simulink model "Test_Comm_and_Motion"  (R2018a)
settings: Solver=FixedStepAuto  StartTime=0.0  StopTime=inf  FixedStep=0.00001  RelTol=1e-3
settings Model: Creator=张紫薇  LastModifiedBy=lenovo

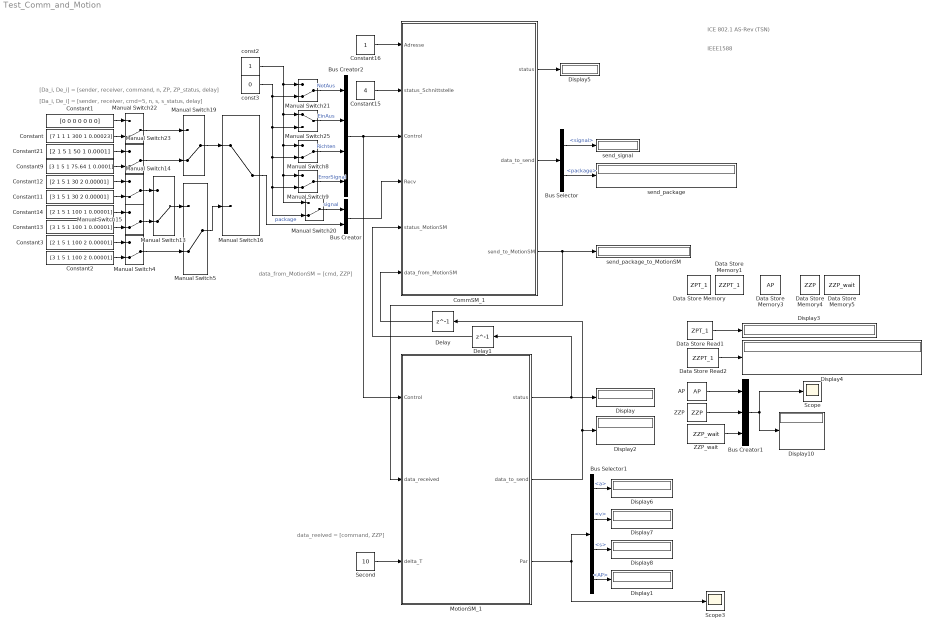
== system Test_Comm_and_Motion ==
  note: IEEE1588
  note: ICE 802.1 AS-Rev (TSN)
  note: data_from_MotionSM = [cmd, ZZP]
  note: [Da_i, De_i] = [sender, receiver, command, n, ZP, ZP_status, delay]
  note: data_reeived = [command, ZZP]
  note: [Da_i, De_i] = [sender, receiver, cmd=5, n, s, s_status, delay]
  AP : DataStoreRead  DataStoreName=AP
  Bus Creator1 : BusCreator  Inputs=3
  Bus Creator : BusCreator  Inputs=2
  Bus Creator2 : BusCreator  Inputs=4
  Bus Selector : BusSelector  OutputSignals=signal,package
  Bus Selector1 : BusSelector  OutputSignals=a,v,s,AP
  CommSM_1 : Subsystem
  Constant : Constant  Value=[7 1 1 1 300 1 0.00023]  OutDataTypeStr=double
  Constant1 : Constant  Value=[0 0 0 0 0 0 0]  OutDataTypeStr=double
  Constant11 : Constant  Value=[3 1 5 1 30 2 0.00001]  OutDataTypeStr=double
  Constant12 : Constant  Value=[2 1 5 1 30 2 0.00001]  OutDataTypeStr=double
  Constant13 : Constant  Value=[3 1 5 1 100 1 0.00001]  OutDataTypeStr=double
  Constant14 : Constant  Value=[2 1 5 1 100 1 0.00001]  OutDataTypeStr=double
  Constant15 : Constant  Value=4  OutDataTypeStr=double
  Constant16 : Constant
  Constant2 : Constant  Value=[3 1 5 1 100 2 0.00001]  OutDataTypeStr=double
  Constant21 : Constant  Value=[2 1 5 1 50 1 0.0001]  OutDataTypeStr=double
  Constant3 : Constant  Value=[2 1 5 1 100 2 0.00001]  OutDataTypeStr=double
  Constant9 : Constant  Value=[3 1 5 1 75.64 1 0.0001]  OutDataTypeStr=double
  Data Store Memory : DataStoreMemory  DataStoreName=ZPT_1  ReadBeforeWriteMsg=warning  WriteAfterWriteMsg=warning  WriteAfterReadMsg=warning  InitialValue=zeros(1,3)  ShowAdditionalParam=off  OutDataTypeStr=double  Dimensions=[1,3]
  Data Store Memory1 : DataStoreMemory  DataStoreName=ZZPT_1  ReadBeforeWriteMsg=warning  WriteAfterWriteMsg=warning  WriteAfterReadMsg=warning  InitialValue=zeros(3,4)  ShowAdditionalParam=off  OutDataTypeStr=double  Dimensions=[3,4]
  Data Store Memory3 : DataStoreMemory  DataStoreName=AP  ReadBeforeWriteMsg=warning  WriteAfterWriteMsg=warning  WriteAfterReadMsg=warning  ShowAdditionalParam=off  OutMin=[0]  OutMax=[100]  OutDataTypeStr=double  Dimensions=1
  Data Store Memory4 : DataStoreMemory  DataStoreName=ZZP  ReadBeforeWriteMsg=warning  WriteAfterWriteMsg=warning  WriteAfterReadMsg=warning  ShowAdditionalParam=off  OutDataTypeStr=double  Dimensions=1
  Data Store Memory5 : DataStoreMemory  DataStoreName=ZZP_wait  ReadBeforeWriteMsg=warning  WriteAfterWriteMsg=warning  WriteAfterReadMsg=warning  ShowAdditionalParam=off  OutDataTypeStr=double  Dimensions=1
  Data Store Read1 : DataStoreRead  DataStoreName=ZPT_1
  Data Store Read2 : DataStoreRead  DataStoreName=ZZPT_1
  Delay : Delay  DelayLength=1
  Delay1 : Delay  DelayLength=1
  Display{,1..8,10} (10 alike) : Display
      Display1 settings: Format=decimal (Stored Integer)
      Display10 settings: Format=decimal (Stored Integer)
      Display8 settings: Format=decimal (Stored Integer)
  Manual Switch{4..5,8..9,13..15,19..23} (12 alike) : ManualSwitch  CurrentSetting=0
  Manual Switch16 : ManualSwitch
  Manual Switch25 : ManualSwitch
  MotionSM_1 : Subsystem
  Scope : Scope
  Scope3 : Scope
  Second : Constant  Value=10
  ZZP : DataStoreRead  DataStoreName=ZZP
  ZZP_wait : DataStoreRead  DataStoreName=ZZP_wait
  const2 : Constant  OutDataTypeStr=boolean
  const3 : Constant  Value=0  OutDataTypeStr=boolean
  send_package : Display
  send_package_to_MotionSM : Display
  send_signal : Display
  wires:
  Manual Switch5/1 -> Manual Switch16/2
  Data Store Read2/1 -> Display4/1
  Manual Switch13/1 -> Manual Switch5/1
  Manual Switch19/1 -> Manual Switch16/1
  Constant3/1 -> Manual Switch4/1
  Delay1/1 -> CommSM_1/5(status_MotionSM)
  Delay/1 -> CommSM_1/6(data_from_MotionSM)
  Constant11/1 -> Manual Switch14/2
  Constant2/1 -> Manual Switch4/2
  const3/1 -> Manual Switch20/2, Manual Switch9/2, Manual Switch8/2, Manual Switch25/2, Manual Switch21/2
  MotionSM_1/1(status) -> Delay1/1, Display/1
  Constant/1 -> Manual Switch22/2
  Data Store Read1/1 -> Display3/1
  Constant1/1 -> Manual Switch22/1
  Bus Selector/1 -> send_signal/1  "<signal>"
  Second/1 -> MotionSM_1/3(delta_T)
  Manual Switch15/1 -> Manual Switch13/2
  Bus Selector/2 -> send_package/1  "<package>"
  Manual Switch4/1 -> Manual Switch5/2
  Constant21/1 -> Manual Switch23/1
  CommSM_1/3(send_to_MotionSM) -> send_package_to_MotionSM/1, MotionSM_1/2(data_received)
  Manual Switch22/1 -> Manual Switch19/1
  Manual Switch14/1 -> Manual Switch13/1
  Bus Selector1/2 -> Display7/1  "<v>"
  Constant14/1 -> Manual Switch15/1
  Constant15/1 -> CommSM_1/2(status_Schnittstelle)
  Bus Selector1/1 -> Display6/1  "<a>"
  Constant12/1 -> Manual Switch14/1
  Constant13/1 -> Manual Switch15/2
  const2/1 -> Manual Switch20/1, Manual Switch9/1, Manual Switch8/1, Manual Switch25/1, Manual Switch21/1
  Constant9/1 -> Manual Switch23/2
  CommSM_1/1(status) -> Display5/1
  MotionSM_1/2(data_to_send) -> Delay/1, Display2/1
  Manual Switch23/1 -> Manual Switch19/2
  Constant16/1 -> CommSM_1/1(Adresse)
  Bus Selector1/3 -> Display8/1  "<s>"
  CommSM_1/2(data_to_send) -> Bus Selector/1
  Manual Switch20/1 -> Bus Creator/1  "signal"
  Manual Switch16/1 -> Bus Creator/2  "package"
  Bus Creator/1 -> CommSM_1/4(Recv)
  MotionSM_1/3(Par) -> Bus Selector1/1, Scope3/1
  ZZP_wait/1 -> Bus Creator1/3
  ZZP/1 -> Bus Creator1/2
  AP/1 -> Bus Creator1/1
  Bus Creator1/1 -> Display10/1, Scope/1
  Bus Selector1/4 -> Display1/1  "<AP>"
  Manual Switch21/1 -> Bus Creator2/1  "NotAus"
  Manual Switch25/1 -> Bus Creator2/2  "EinAus"
  Manual Switch8/1 -> Bus Creator2/3  "Richten"
  Manual Switch9/1 -> Bus Creator2/4  "ErrorSignal"
  Bus Creator2/1 -> MotionSM_1/1(Control), CommSM_1/3(Control)

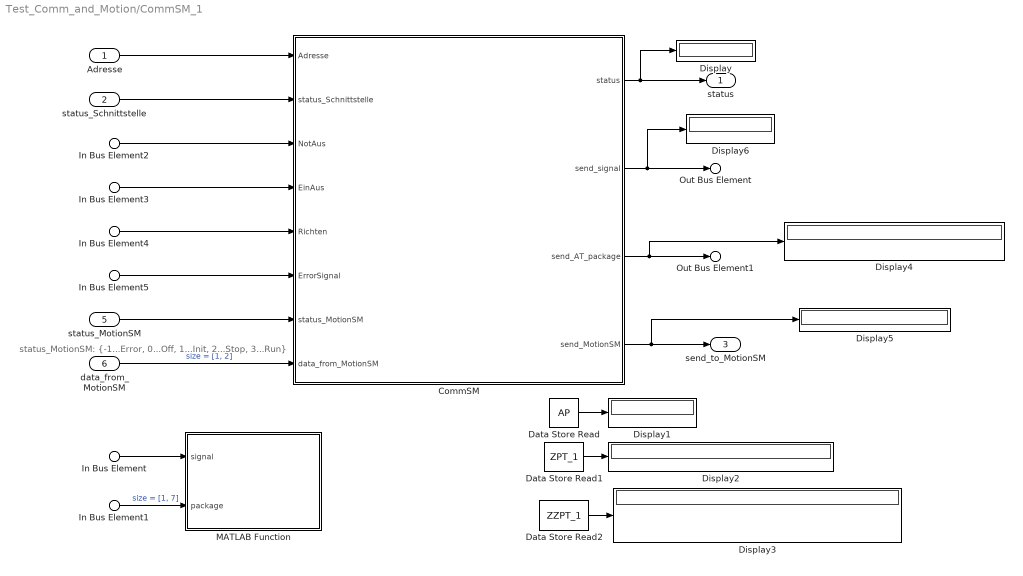
== system Test_Comm_and_Motion/CommSM_1 ==
  note: status_MotionSM: {-1...Error, 0...Off, 1...Init, 2...Stop, 3...Run}
  Adresse : Inport  OutDataTypeStr=double  PortDimensions=1
  status_Schnittstelle : Inport  Port=2  OutDataTypeStr=double  PortDimensions=1
  In Bus Element2 : Inport  Port=3  PortName=Control  Element=NotAus
  In Bus Element3 : Inport  Port=3  PortName=Control  Element=EinAus
  In Bus Element4 : Inport  Port=3  PortName=Control  Element=Richten
  In Bus Element5 : Inport  Port=3  PortName=Control  Element=ErrorSignal
  In Bus Element : Inport  Port=4  PortName=Recv  Element=signal
  In Bus Element1 : Inport  Port=4  PortName=Recv  Element=package
  status_MotionSM : Inport  Port=5  OutDataTypeStr=double  PortDimensions=1
  data_from_MotionSM : Inport  Port=6  OutDataTypeStr=double  PortDimensions=2
  CommSM : Stateflow chart  TreatAsAtomicUnit=on
  Data Store Read : DataStoreRead  DataStoreName=AP
  Data Store Read1 : DataStoreRead  DataStoreName=ZPT_1
  Data Store Read2 : DataStoreRead  DataStoreName=ZZPT_1
  Display{,1..6} (7 alike) : Display
  MATLAB Function : MATLAB Function  TreatAsAtomicUnit=on
  status : Outport  OutDataTypeStr=double  PortDimensions=1
  Out Bus Element : Outport  Port=2  PortName=data_to_send  Element=signal
  Out Bus Element1 : Outport  Port=2  PortName=data_to_send  Element=package
  send_to_MotionSM : Outport  Port=3
  wires:
  In Bus Element2/1 -> CommSM/3(NotAus)
  In Bus Element3/1 -> CommSM/4(EinAus)
  In Bus Element4/1 -> CommSM/5(Richten)
  In Bus Element5/1 -> CommSM/6(ErrorSignal)
  status_Schnittstelle/1 -> CommSM/2(status_Schnittstelle)
  In Bus Element/1 -> MATLAB Function/1(signal)
  In Bus Element1/1 -> MATLAB Function/2(package)  "size = [1, 7]"
  data_from_MotionSM/1 -> CommSM/8(data_from_MotionSM)  "size = [1, 2]"
  status_MotionSM/1 -> CommSM/7(status_MotionSM)
  Adresse/1 -> CommSM/1(Adresse)
  CommSM/1(status) -> Display/1, status/1
  CommSM/3(send_AT_package) -> Out Bus Element1/1, Display4/1
  CommSM/4(send_MotionSM) -> Display5/1, send_to_MotionSM/1
  CommSM/2(send_signal) -> Out Bus Element/1, Display6/1
  Data Store Read/1 -> Display1/1
  Data Store Read1/1 -> Display2/1
  Data Store Read2/1 -> Display3/1

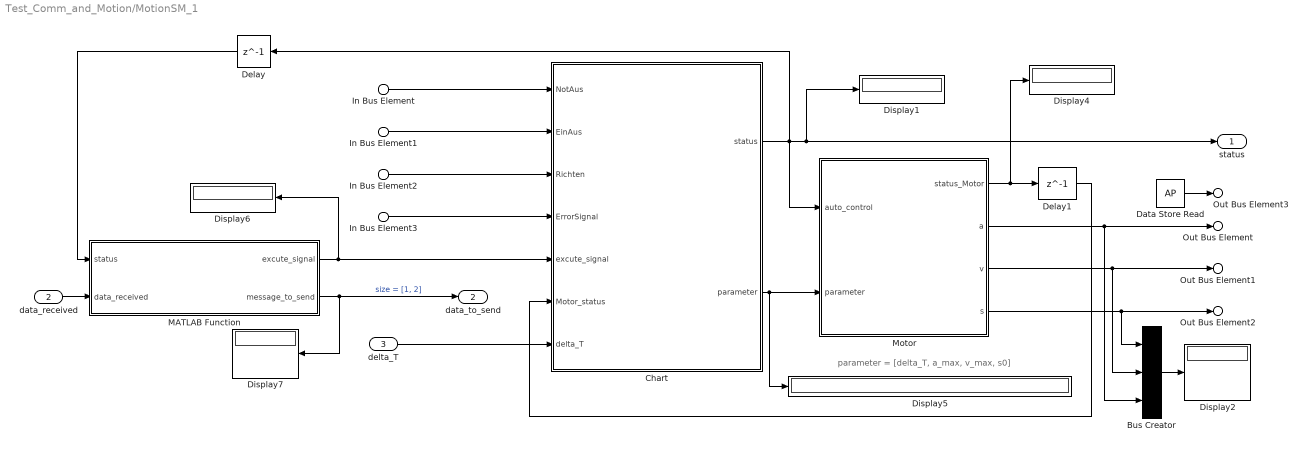
== system Test_Comm_and_Motion/MotionSM_1 ==
  note: parameter = [delta_T, a_max, v_max, s0]
  In Bus Element : Inport  PortName=Control  Element=NotAus
  In Bus Element1 : Inport  PortName=Control  Element=EinAus
  In Bus Element2 : Inport  PortName=Control  Element=Richten
  In Bus Element3 : Inport  PortName=Control  Element=ErrorSignal
  data_received : Inport  Port=2  OutDataTypeStr=double  PortDimensions=2
  delta_T : Inport  Port=3
  Bus Creator : BusCreator  Inputs=3
  Chart : Stateflow chart  TreatAsAtomicUnit=on
  Data Store Read : DataStoreRead  DataStoreName=AP
  Delay : Delay  DelayLength=1
  Delay1 : Delay  DelayLength=1
  Display{1..2,4..7} (6 alike) : Display
  MATLAB Function : MATLAB Function  TreatAsAtomicUnit=on
  Motor : Subsystem
  status : Outport
  data_to_send : Outport  Port=2  OutDataTypeStr=double  PortDimensions=2
  Out Bus Element : Outport  Port=3  PortName=Par  Element=a
  Out Bus Element1 : Outport  Port=3  PortName=Par  Element=v
  Out Bus Element2 : Outport  Port=3  PortName=Par  Element=s
  Out Bus Element3 : Outport  Port=3  PortName=Par  Element=AP
  wires:
  Chart/1(status) -> Motor/1(auto_control), Delay/1, Display1/1, status/1
  In Bus Element1/1 -> Chart/2(EinAus)
  In Bus Element/1 -> Chart/1(NotAus)
  In Bus Element2/1 -> Chart/3(Richten)
  In Bus Element3/1 -> Chart/4(ErrorSignal)
  Motor/1(status_Motor) -> Display4/1, Delay1/1
  data_received/1 -> MATLAB Function/2(data_received)
  Delay1/1 -> Chart/6(Motor_status)
  MATLAB Function/1(excute_signal) -> Chart/5(excute_signal), Display6/1
  MATLAB Function/2(message_to_send) -> Display7/1, data_to_send/1  "size = [1, 2]"
  delta_T/1 -> Chart/7(delta_T)
  Motor/2(a) -> Bus Creator/3, Out Bus Element/1
  Motor/3(v) -> Bus Creator/2, Out Bus Element1/1
  Motor/4(s) -> Bus Creator/1, Out Bus Element2/1
  Chart/2(parameter) -> Motor/2(parameter), Display5/1
  Delay/1 -> MATLAB Function/1(status)
  Data Store Read/1 -> Out Bus Element3/1
  Bus Creator/1 -> Display2/1

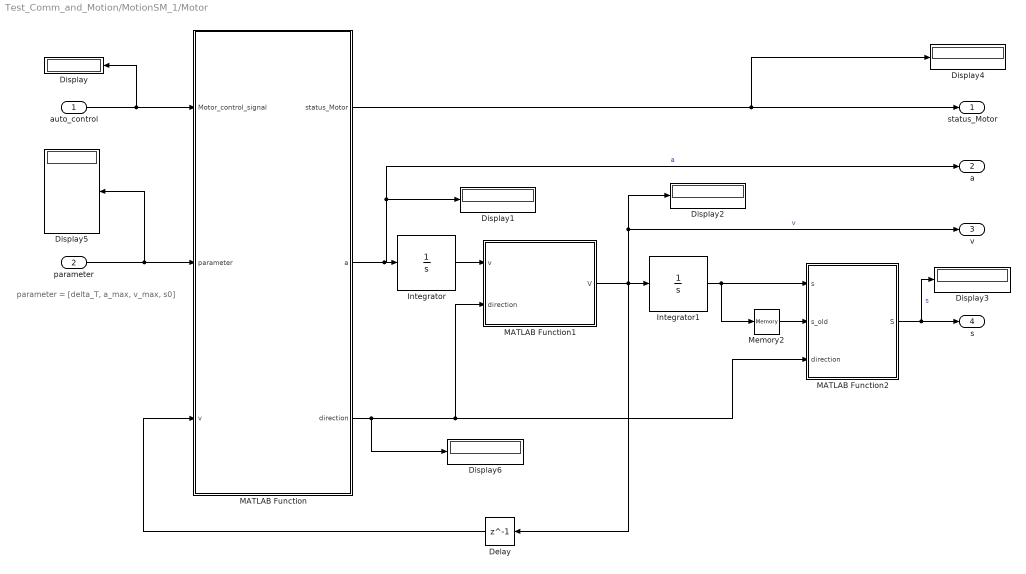
== system Test_Comm_and_Motion/MotionSM_1/Motor ==
  note: parameter = [delta_T, a_max, v_max, s0]
  auto_control : Inport
  parameter : Inport  Port=2
  Delay : Delay  DelayLength=1
  Display{,1..6} (7 alike) : Display
  Integrator : Integrator
  Integrator1 : Integrator
  MATLAB Function : MATLAB Function  TreatAsAtomicUnit=on
  MATLAB Function1 : MATLAB Function  TreatAsAtomicUnit=on
  MATLAB Function2 : MATLAB Function  TreatAsAtomicUnit=on
  Memory2 : Memory
  status_Motor : Outport
  a : Outport  Port=2
  v : Outport  Port=3
  s : Outport  Port=4
  wires:
  Integrator/1 -> MATLAB Function1/1(v)
  Integrator1/1 -> MATLAB Function2/1(s), Memory2/1
  auto_control/1 -> Display/1, MATLAB Function/1(Motor_control_signal)
  MATLAB Function/1(status_Motor) -> Display4/1, status_Motor/1
  parameter/1 -> Display5/1, MATLAB Function/2(parameter)
  MATLAB Function/2(a) -> a/1, Display1/1, Integrator/1  "a"
  MATLAB Function1/1(V) -> Display2/1, v/1, Delay/1, Integrator1/1  "v"
  MATLAB Function/3(direction) -> MATLAB Function1/2(direction), MATLAB Function2/3(direction), Display6/1
  MATLAB Function2/1(S) -> Display3/1, s/1  "s"
  Memory2/1 -> MATLAB Function2/2(s_old)
  Delay/1 -> MATLAB Function/3(v)

== matlab function Test_Comm_and_Motion/MotionSM_1/MATLAB Function ==
  data: status input double size=1; excute_signal output boolean size=1; message_to_send output double size=2; data_received input double size=2; ZZP_wait data_store_memory size=1; AP data_store_memory; ZZP data_store_memory
%data_received / message_to_send = [cmd, ZZP]
%cmd:  1...setP, 2...getP, 3...excP

function [excute_signal, message_to_send] = message_analysis(status, data_received)

global ZZP_wait
global AP
global ZZP

excute_signal = false;

cmd = data_received(1);
message_to_send = [0, 0]';

switch cmd
    case 1      %setP
        excute_signal = false;
        if ((status >= 1) && (status <= 3))
            ZZP_wait = data_received(2);
            message_to_send = [2, ZZP_wait]';
        end
        
    case 3      %excP
        excute_signal = true;
        if ((ZZP == AP) && (status == 2) && (ZZP~=ZZP_wait))
            ZZP = ZZP_wait;
        end
end
end

== matlab function Test_Comm_and_Motion/MotionSM_1/Motor/MATLAB Function ==
  settings: updateMethod=DISCRETE
  data: status_Motor output boolean size=1; Motor_control_signal input double size=1; parameter input double size=4; v input double size=1; a output double size=1; direction output double size=1; AP data_store_memory; ZZP data_store_memory
function [status_Motor, a, direction]= Motor(Motor_control_signal, parameter, v)

%delta_T = parameter(1);
a_max = abs(parameter(2));
v_max = abs(parameter(3));
s0 = parameter(4);
direction = 0;
a = 0;

s_a = 0.5 * v_max * v_max / a_max;
a_bremsen = 100000;     % 100 m/s^2

global AP
global ZZP

switch Motor_control_signal
    case {-1, 0}            %Error & Off
        if v > 0
            a = -a_bremsen;
            direction = 1;
        elseif v < 0
            a = a_bremsen;
            direction = -1;
        else
            a = 0;
            direction = 0;
        end
             
    case 1                  %Init
        if (AP > 0)
            direction = s0;
            if ((ZZP - AP) < (-s_a)) && (v > (-v_max))
                a = -a_max;
            elseif ((ZZP - AP) >= (-s_a)) && (ZZP < AP) && (v < 0)
                a = a_max;
            else
                a = 0;
            end
        else
            a = 0;
            AP = 0;
        end
        
    case 2                  %Stop
        if (v > 0)
            a = -a_max;
            direction = 1;
        elseif (v < 0)
            a = a_max;
            direction = -1;
        else
            a = 0;
            direction = 0;
        end
        
    case 3                  %run
        direction = s0;
        if (s0 > 0)   %forward
            %v_control(2) = s0;
            if ((ZZP - AP) > s_a) && (v < v_max)
                a = a_max;
            elseif ((ZZP - AP) <= s_a) && (ZZP > AP) && (v > 0)
                a = -a_max;
            else
                a = 0;
            end
        end
        if (s0 < 0)    %backward
            if ((ZZP - AP) < (-s_a)) && (v > (-v_max))
                a = -a_max;
            elseif ((ZZP - AP) >= (-s_a)) && (ZZP < AP) && (v < 0)
                a = a_max;
            else
                a = 0;
            end
        end
end
        
%status_Motor: false...Stopped, true...Running
if (a == 0) && (v == 0)
    status_Motor = false;
else
    status_Motor = true;
end

end

== stateflow chart Test_Comm_and_Motion/MotionSM_1/Chart ==
  state Off
    entry: status=0;
  state Init
    entry: status=1; parameter=Par_1(delta_T);
  state On
    state Stop
      entry: status=2;
    state Run
      entry: status=3;
    (default) -> Stop
    Stop -> Run : [excute_signal==1 && ZZP~=AP && Motor_status == 0]
        | {parameter=Par(delta_T)}
    Run -> Stop : [ZZP==AP && ~Motor_status]
  state Error
    entry: status=-1;
  (default) -> Off
  Init -> Off [order 1] : [~EinAus]
  Off -> Init [order 2] : [EinAus && ~ NotAus]{parameter=[delta_T,0,0,0]'}
  Init -> Error [order 2] : [Motor_status==-1 || NotAus || ErrorSignal]
  Off -> Error [order 1] : [EinAus && (ErrorSignal || NotAus)]
  Error -> Off [order 1] : [~EinAus]
  On -> Off [order 1] : [~EinAus]
  Error -> Init [order 2] : [Richten]{parameter=[delta_T,0,0,0]'}
  Init -> On [order 3] : [AP==0]{parameter=[delta_T,0,0,0]'}
  On -> Error [order 2] : [Motor_status==-1 || NotAus || ErrorSignal]
  data: par function_output double size=4; delta_t function_input double size=1; par function_output double size=4; delta_t function_input double size=1; NotAus input boolean size=1; EinAus input boolean size=1; Richten input boolean size=1; ErrorSignal input boolean size=1; excute_signal input boolean size=1; Motor_status input boolean size=1; status output double size=1 =0; ZZP data_store_memory; ZZP_wait data_store_memory; parameter output double size=4; AP data_store_memory size=1; delta_T input double size=1
  function par = Par_1(delta_t):
    | function par = Par_1(delta_t)
    | 
    | global ZZP
    | global ZZP_wait
    | global AP
    | 
    | % delta_T = 10 s
    | ZZP = 0;
    | ZZP_wait = 0;
    | s0 = ZZP - AP;
    | a_max = 100;        % 1 m/s^2
    | v_max = 1;
    | %v_max = 0.5 * a_max * (delta_t - sqrt(delta_t*delta_t - 4*abs(s0)/a_max));   	% mm/s
    | 
    | par = [delta_t, a_max, v_max, s0]';
    | end
  function par = Par(delta_t):
    | function par = Par(delta_t)
    | 
    | global ZZP
    | global AP
    | 
    | s0 = ZZP - AP;
    | a_max = 1000;       % 1 m/s^2
    | v_max = 0.5 * a_max * (delta_t - sqrt(delta_t*delta_t - 4*abs(s0)/a_max));  % mm/s
    | 
    | par = [delta_t, a_max, v_max, s0]';
    | end

== matlab function Test_Comm_and_Motion/MotionSM_1/Motor/MATLAB Function1 ==
  settings: updateMethod=DISCRETE
  data: V output; v input; direction input double size=1; AP data_store_memory; ZZP data_store_memory
function V = v_conrol(v, direction)

global AP
global ZZP

if direction > 0
    if ((v < 0) || (AP >= ZZP))
        V = 0;
    else
        V = v;
    end
elseif direction < 0
    if v > 0 || (AP <= ZZP)
        V = 0;
    else
        V = v;
    end
else
    V = 0;
end
end

== matlab function Test_Comm_and_Motion/MotionSM_1/Motor/MATLAB Function2 ==
  settings: updateMethod=DISCRETE
  data: s input; s_old input; S output; direction input double size=1; AP data_store_memory; ZZP data_store_memory
function S = s_control(s, s_old, direction)

global AP
global ZZP

if direction > 0
    if (AP + s - s_old) < ZZP
        S = s;
        AP = AP + s - s_old;
    else
        S = s_old;
        AP = ZZP;
    end
elseif direction < 0
    if (AP + s - s_old) > ZZP
        S = s;
        AP = AP + s - s_old;
    else
        S = s_old;
        AP = ZZP;
    end
else
    S = s_old;
end

end

== stateflow chart Test_Comm_and_Motion/CommSM_1/CommSM ==
  state Init
    entry: 	status=1;
    send_AT_package=[Adresse, zeros(1,5)];
    send_signal=false;
    send_MotionSM=[0,0];
  state Aus
    entry: status=0;
  state Ein
    note: % Protokoll
        | % SummenTelegramm = [HDR, SDT, END]
        | %HDR: header, SDT: Summen-Daten-Telegramm, END: Ender
        |
        | % SDT = [SDT_7, SDT_1, SDT_2, SDT_3]
        | % SDT_i = [Da_i, De_i]
        | %Da: Data, De: Delay
        | %i...{1,2,3,7} %7...GSM, 1-3...CommSM1-3
        |
        | % Da_i = [sender, receiver, cmd, N, ZP, ZP_status]
        | %sender,receiver...{1,2,3,7,255} %255...Broadcast
        | %cmd: 1...addP, 2...getP, 3...setS, 4...getS
        | %ZP_status: 0...none, 1...wait, 2...active, 3...done, 4...error
        |
        | % Da_i = [sender, receiver, cmd, N, s , s _status]
        | %cmd: 5 ...negO
        | % s _status: 0...none, 1...negotiation, 2...excute, 3...done
    state Free
      entry:	status=2;
      send_signal=false;
      send_AT_package=zeros(1,6);
    state SkillRequest
      entry:	status=3;
      send_AT_package=[Adresse, 7, 2, ZPT_1(1), ZPT_1(2), ZPT_1(3)];
      % AT=[CommSM, GSM, getP, n, ZP, wait];
      send_signal=true;
    state send_AT_2_GSM
      entry:	status=13;
      send_AT_package=[Adresse, 7, 3, ZPT_1(1), ZPT_1(2), ZPT_1(3)];
      %AT=[CommSM, GSM, setS, n, ZP, done];
      send_signal=true;
    state activ
      entry:	status=4;
      ZPT_1(3)=2;	% status='active'
      send_AT_package=[Adresse, 7, 3, ZPT_1(1), ZPT_1(2), ZPT_1(3)];
      % AT=[CommSM, GSM, setS, n, ZP, activ];
      send_signal=true;
    state Arrival
      entry:	status=12;
      ZPT_1(3)=3;
    state check_ZP
      entry: 	status=5;
      s=checkZP(ZZP_old, Adresse);
      % s-range: [0, 100], ZZP_old: ZZP for last Loop
      send_AT_package=[Adresse, 255, 5, ZPT_1(1), s, 1];
      % AT=[CommSM, Broadcast, negO, n, s, nego];
      send_signal=true;
    state MotionSM
      entry:	status=11;
      send_MotionSM=[3, ZZPT_1(Adresse,2)];	%excute ZZP
    state Nego_wait
      entry: 	status=6;
    state Wait_excution
      entry:	status=10;
      send_AT_package=[Adresse, 255, 5, ZPT_1(1), ZZPT_1(Adresse, 4), 2];
      %AT=[CommSM, Broadcast, negO, n, s, excu];
      send_signal=true;
      send_MotionSM=[1, ZZPT_1(Adresse,2)]; %set ZZP
    state status_excution
      entry: 	status=9;
      ZZPT_1(Adresse,4)=2; %excu
    state s_Compair
      entry: 	status=7; s_new=s_compair(Adresse);
    state ZZP_new
      entry:	status=8;
      ZZPT_1(Adresse,3)=s_new;
      ZZPT_1(Adresse,2)=AP+(ZPT_1(2)-AP)*(s_new/100);
    (default) -> Free
    (junction 118) -> Free
    send_AT_2_GSM -> (junction 118) : {send_signal=false; ZPT_1=zeros(1,3)';}
    Free -> SkillRequest : %Datei von GSM empfangen
        | [ZPT_1(1)~=0]
    SkillRequest -> activ : %status="wait" && MotionSM kein Fehler
        | [ZPT_1(3)==1 && status_MotionSM>=1]{send_signal=false;}
    (junction 77) -> send_AT_2_GSM
    Arrival -> (junction 77)
    (junction 121) -> (junction 77)
    MotionSM -> Arrival [order 1] : % ZP == ZZP -> wait until ZP == AP
        | [ZPT_1(2)==AP && ZZPT_1(Adresse,2)==AP && status_MotionSM ==2]
        | {ZZPT_1=zeros(3,4); send_MotionSM=zeros(1,2)}
    activ -> (junction 99) : [ZPT_1(3)==2]{send_signal=false;}
    (junction 116) -> (junction 99)
    (junction 99) -> check_ZP
    MotionSM -> (junction 116) [order 2] : % ZP~=ZZP = ZZP = ZZP -> cycle
        | [ZPT_1(2)~=ZZPT_1(Adresse,2)]
        | {ZZP_old=ZZPT_1(Adresse,2); ZZPT_1=zeros(3,4);}
    (junction 146) -> MotionSM : [status_MotionSM==2] % Motor stoped
    check_ZP -> Nego_wait : {s=0; send_signal=false;}
    (junction 125) -> (junction 146) : % ZZP received from MotionSM
        | [data_from_MotionSM(1)==2 && data_from_MotionSM(2)==ZZPT_1(Adresse,2)]{ZZP_old=0;}
    Wait_excution -> (junction 125) : [ZZPT_1(1,4)==2 && ZZPT_1(2,4)==2 && ZZPT_1(3,4)==2]{send_signal=false;}
    Nego_wait -> (junction 121) [order 1] : [ZPT_1(3)==3] % ZP = AP
    Nego_wait -> (junction 134) [order 2] : [ZPT_1(3)==2] % ZP "activ"
    status_excution -> Wait_excution : [status_MotionSM>=2]  % 2 or 3
    (junction 134) -> s_Compair : %ZZPT erfüllt
        | [ZZPT_1(1,1)==1 && ZZPT_1(2,1)==1 && ZZPT_1(3,1)==1 && ZZPT_1(1,1)~=0]
    s_Compair -> (junction 79)
    (junction 66) -> status_excution : {s_new=0;}
    (junction 79) -> (junction 66) [order 2] : [s_new>=ZZPT_1(Adresse,3)]
    (junction 79) -> ZZP_new [order 1] : [s_new<ZZPT_1(Adresse,3)]
    ZZP_new -> (junction 66)
  state Error
    entry: status=-1;
  (default) -> Aus
  Aus -> Init : [EinAus && ~NotAus && ~ErrorSignal]
  Init -> Aus [order 1] : [~EinAus]
  Init -> Error [order 2] : [NotAus]
  Error -> Aus [order 1] : [~EinAus]
  Ein -> Aus [order 1] : [~EinAus]
  Error -> Init [order 2] : [Richten && ~NotAus && ~ErrorSignal]
  Init -> Ein [order 3] : [status_Schnittstelle==4]{send_signal=false;}
  Ein -> Error [order 2] : [NotAus]
  data: zzp_old function_input double size=1; S function_output; adress function_input double size=1; S_new function_output double size=1; nr function_input double size=1; Adresse input double size=1; status_Schnittstelle input double size=1; NotAus input boolean size=1; EinAus input boolean size=1; Richten input boolean size=1; ErrorSignal input boolean size=1; status output double size=1; send_signal output boolean size=1 =false; send_AT_package output double size=[1,6] =zeros(1,6); status_MotionSM input double size=1; data_from_MotionSM input double size=[1,2]; ZPT_1 data_store_memory; ZZPT_1 data_store_memory; AP data_store_memory; s local double size=1 =0; s_new local double size=1 =0; send_MotionSM output double size=[1,2] =zeros(1,2); ZZP_old local double size=1 =0
  function S = checkZP(zzp_old, adress):
    | %ZPT_1 = [ZP_Nr., ZP, status]
    | %status: {0...none, 1...wait, 2...active, 3...done, 4...error}
    | 
    | %ZZPT_1(CommSM_i,:) = [ZP-Nr., ZZP, s%, status]
    | %status: {0...none, 1...negotiation, 2...excution, 3...done}
    | 
    | function S = checkZP(zzp_old, adress)
    | %1. prüfen, ob ZP unter begrenzte Bedienung erreichbar ist
    |         %Ja     --> ZZP = ZP
    |         %Nein   --> neuen ZZP erzeugen
    | %2. neu ausgerechnete ZZP in der ZZP Tabelle einschreiben
    |  
    | global AP
    | global ZPT_1
    | global ZZPT_1
    | 
    | a_max = 1000;   % mm/s^2
    | v_max = 1000;   % mm/s
    | d_T = 10;    % s
    | 
    | s_max = a_max*d_T*d_T/4;
    | if zzp_old <= 0             %last ZZP to arrive. After the Motor is started, ZZP_old = ZZP, ZZPT = zeros(3,4);
    |     s0 = ZPT_1(2) - AP;     %ZP - AP
    | else
    |     s0 = ZPT_1(2) - zzp_old;    %excist last ZZP
    | end
    | 
    | if abs(s0) <= s_max
    |     S = 100;                    % 100% erreichbar
    | elseif abs(s0) > 0 && abs(s0) < 100
    |     S = abs(100*s_max/s0);      % s% s: [0, 100]
    |     S = fix(1000*S)/1000;       % Genauigkeit = 10000*0.001%=0.1 mm
    | else
    |     S = 0;                      % ZP = AP, Achse keine Bewegung
    | end
    | 
    | %ZZP-Tabelle erfüllen
    | if zzp_old <= 0
    |     ZZP_new = AP + s0*S/100;        %neue ZZP in der ZZP-Tabelle einschreiben
    | else
    |     ZZP_new = zzp_old+s0*S/100;
    | end
    | 
    | if S == 0
    |     %ZZPT_1(nr,:) = [ZPT_1(1), ZZP_new, s, 3];
    |     ZPT_1(3) = 3;
    | else
    |     ZZPT_1(adress,:) = [ZPT_1(1), ZZP_new, S, 1];
    | end
    | 
    | end
  function S_new = s_compair(nr):
    | function S_new = s_compair(nr)
    | 
    | global ZZPT_1
    | 
    | s_ = ZZPT_1(:,3);
    | 
    | S_new = s_(nr);          % CommSM_me
    | 
    | for i = 1:3                         % s==0 --> s=100
    |     if i ~= nr && s_(i)== 0
    |         s_(i) = 100;
    |     end
    | end
    | 
    | s_min = min(s_);
    | if S_new > s_min
    |     S_new = s_min;
    | end
    | 
    | end

== matlab function Test_Comm_and_Motion/CommSM_1/MATLAB Function ==
  data: signal input boolean size=1; package input double size=[1,7]; ZPT_1 data_store_memory; ZZPT_1 data_store_memory
%Protokoll
%SummenTelegramm = [HDR, SDT, END]
	%HDR: header,	SDT: Summen-Daten-Telegramm,    END: Ender

%SDT = [SDT_7, SDT_1, SDT_2, SDT_3]
%SDT_i = [Da_i, De_i]
	%Da: Data, De: Delay
	%i...{1,2,3,7}	%7...GSM, 1-3...CommSM1-3

%Da_i = [sender, receiver, cmd, N, ZP, ZP_status]
	%sender,receiver...{1,2,3,7,255}	%255...Broadcast
	%cmd: 111...addP, 112...getP, 113...setS, 114...getS
	%ZP_status: 0...none, 1...wait, 2...active, 3...done, 4...error

%Da_i = [sender, receiver, cmd, N, s, s_status]
	%cmd: 115...negO
	%s_status: 0...none, 1...negotiation, 2...excute, 3...done


% Hier werden nur die Befehlen, die ZPT oder ZZPT behandeln möchte, werden behandelt.
function receive_AT(signal, package)

global ZPT_1
global ZZPT_1

if signal
    switch package(1)  % from GSM
        case 7
            if (package(3) == 111)   % cmd == 'add Position'
                if ZPT_1(1) == 0
                    ZPT_1 = package(4:6)';    %[n, ZP, status='wait']
                end
            end
            
        case {2,3}      % from CommSM_2 or CommSM_3
            if package(3) == 115      % negotiation
                switch package(6)
                    case 1      % nego
                        ZZPT_1(package(1),:) = [package(4), 0, package(5:6)];     % [n, ZP, s%, status='nego']
                    case 2      % excu
                        if ZZPT_1(package(1),4) == 1
                            ZZPT_1(package(1),4) = package(6);
                        end
                end
            end
    end
end

end
